simulink model "walkingRobotRL3D"  (R2020b)
settings: Solver=ode23t  StartTime=0.0  StopTime=Tf  RelTol=1e-2  EnableMultiTasking=on
PreLoadFcn:
  | robotParametersRL
undefined symbols (not defined in the file): agent, ankleD_pitch_jointMAX, ankleD_pitch_jointMIN, ankleD_roll_jointMAX, ankleD_roll_jointMIN, ankleI_pitch_jointMAX, ankleI_pitch_jointMIN, ankleI_roll_jointMAX, ankleI_roll_jointMIN, getSampleTime, height_plane, hipD_pitch_jointMAX, hipD_pitch_jointMIN, hipD_roll_jointMAX, hipD_roll_jointMIN, hipI_pitch_jointMAX, hipI_pitch_jointMIN, hipI_roll_jointMAX, hipI_roll_jointMIN, init_angs_L, init_angs_R, init_height, joint_damping, joint_limit_damping, joint_limit_stiffness, joint_stiffness, kneeD_jointMAX, kneeD_jointMIN, kneeI_jointMAX, kneeI_jointMIN, lower_leg_I0, lower_leg_length, lower_leg_mass, lower_leg_x, lower_leg_y, muscle_nominal_length, p10_ankleD_roll, plane_x, plane_y, regulator_type, tau, Tf, torso_height, torso_length, torso_offset_x, torso_offset_z, torso_width, torso_x, torso_y, torso_z, Ts, upper_leg_I0, upper_leg_length, upper_leg_mass, upper_leg_x, upper_leg_y, v10_ankleD_pitch, v10_ankleD_roll, v10_ankleI_pitch, v10_ankleI_roll ... (+41)
libraries: sm_lib x222, simulink x183, nesl_utility x130, walkingRobotUtils x69, rllib x2
(part 1 of 24)
settings Model: Creator=scastro  LastModifiedBy=eri53
settings SolverCC: ZeroCrossAlgorithm=Adaptive
settings DataIOCC: SaveOutput=off  SignalLogging=off  DSMLogging=off  SaveTime=off  ReturnWorkspaceOutputs=off  OutputTimes=0:0.01:10  Refine=2
settings OptimizationCC: LifeSpan=inf
settings DebuggingCC: MaxConsecutiveZCsMsg=warning  IgnoredZcDiagnostic=none  AllowSymbolicDim=off  SFUnexpectedBacktrackingDiag=warning  SFNoUnconditionalDefaultTransitionDiag=warning  SFExecutionAtInitializationDiag=none  UnitsInconsistencyMsg=none  ArithmeticOperatorsInVariantConditions=warning
settings SFSimCC: SimUseLocalCustomCode=off  CustomCodeUndefinedFunction=UseInterfaceOnly
settings RTWCC: RTWUseLocalCustomCode=off
settings CodeAppCC: StateflowObjectComments=on
settings GRTTargetCC: TargetLangStandard=C89/C90 (ANSI)
settings ConfigComp: CovMetricSettings=dw  CovSaveCumulativeToWorkspaceVar=on  CovSaveSingleToWorkspaceVar=on  CovExternalEMLEnable=off  CovSFcnEnable=off
settings SimscapeCC: SimscapeNormalizeSystem=off  SimscapeLogOpenViewer=on  SimscapeLogLimitData=off  SimscapeLogDataHistory=10000
settings ConfigurationSet: Description=SimMechanics 2G
settings DiagnosticsConfigSet: SimMechanicsRigidlyBoundBlock=none
settings ExplorerConfigSet: InternalSimMechanicsExplorerSettings="<ExplorerConfiguration><canonicalview>default</canonicalview><AnimationSetting><BasePlaybackSpeed>1.0</BasePlaybackSpeed><PlaybackSpeedFactor>1.0</PlaybackSpeedFactor></AnimationSetting><TilePanel><TileInfo><Tiles Columns=\"1\" Count=\"1\" Rows=\"1\"><Column Weight=\"1\"/><Row Weight=\"1\"/><Tile Height=\"1\" Width=\"1\" X=\"0\" Y=\"0\"/></Tiles></TileInfo><SceneInfo><SceneViewer><BGColor><R>0.60000002384185791</R><G>0.60000002384185791</G><B>0.60000002384185791</B></BGColor><Camera><DoPerspective>off</DoPerspective><Position><X>8.85055587658612453</X><Y>-7.80751437224638067</Y><Z>7.43266399890212259</Z></Position><Center><X>2.77794058095722196</X><Y>0.225775596241813759</Y><Z>-0.252680675913408259</Z></Center><Up><X>-0.335329266167064488</X><Y>0.506481739462631531</Y><Z>0.79437430147428989</Z></Up><ViewLimDist>1</ViewLimDist><YLim>1.59312668712743077</YLim><XLim>2.57988071665439289</XLim></Camera></SceneViewer></SceneInfo></TilePanel><MechEditorPanel><Cameras/><GfxPanelCameraMap/><VideoCreator><PlaybackSpeedRatio>1.0</PlaybackSpeedRatio><FrameRate>30</FrameRate><VideoFormat>Motion JPEG AVI</VideoFormat><FrameSize>auto</FrameSize></VideoCreator></MechEditorPanel></ExplorerConfiguration>"

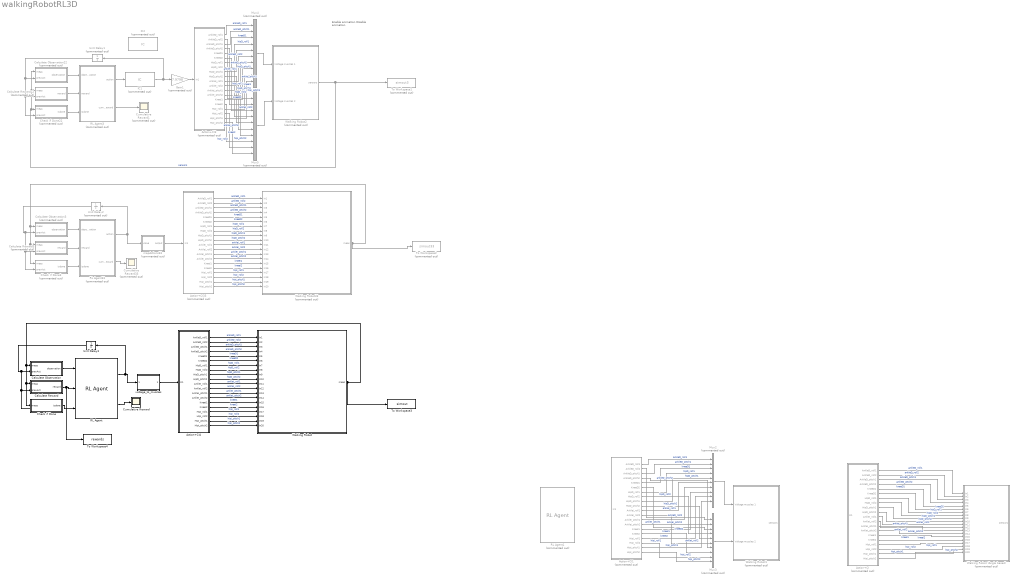
== system walkingRobotRL3D ==
  note: Enable animation
      |
      | Disable animation
  Action+CI : Subsystem  Commented=on
  Action+CI1 : Subsystem  Commented=on
  Action+CI3 : Subsystem  Commented=on
  Action+CI33 : Subsystem  Commented=on
  Action+CI4 : Subsystem
  Calculate Observation : Subsystem
  Calculate Observation22 : Subsystem  Commented=on
  Calculate Observation3 : Subsystem  Commented=on
  Calculate Reward : Subsystem
  Calculate Reward22 : Subsystem  Commented=on
  Calculate Reward3 : Subsystem  Commented=on
  Check if Done : Subsystem
  Check if Done22 : Subsystem  Commented=on
  Check if Done3 : Subsystem  Commented=on
  Cumulative Reward : Scope
  Cumulative Reward1 : Scope  Commented=on
  Cumulative Reward33 : Scope  Commented=on
  Gain1 : Gain  Commented=on  Gain=7.9798
  IC1 : InitialCondition  Commented=on  Value=[v10_ankleD_roll v20_ankleD_roll v10_ankleD_pitch v20_ankleD_pitch v10_kneeD v20_kneeD v10_hipD_roll v20_hipD_roll v10_hipD_pitch v20_hipD_pitch v10_ankleI_roll v20_ankleI_roll v10_ankleI_pitch v20_ankleI_pitch v10_kneeI v20_kneeI v10_hipI_roll v20_hipI_roll v10_hipI_pitch v20_hipI_pitch]'
  IC2 : InitialCondition  Commented=on  Value=(1/7.9798)*[v10_ankleD_roll v20_ankleD_roll v10_ankleD_pitch v20_ankleD_pitch v10_kneeD v20_kneeD v10_hipD_roll v20_hipD_roll v10_hipD_pitch v20_hipD_pitch v10_ankleI_roll v20_ankleI_roll v10_ankleI_pitch v20_ankleI_pitch v10_kneeI v20_kneeI v10_hipI_roll v20_hipI_roll v10_hipI_pitch v20_hipI_pitch]'
  Mux{2..5} (4 alike) : Mux  Commented=on  Inputs=10
  RL Agent : rllib/RL Agent  Agent=agent  ProvideReward=on  ProvideIsDone=on  ProvideCumRwd=on  TreatAsDirectFeedthrough=on  CollectLoggedSignals=on  CollectModelStates=on
  RL Agent1 : rllib/RL Agent  Commented=on  Agent=agent  ProvideReward=on  ProvideIsDone=on  ProvideCumRwd=on  TreatAsDirectFeedthrough=on  CollectLoggedSignals=on  CollectModelStates=on
      settings: SourceProductName=Reinforcement Learning
  RL Agent3 : Subsystem  Commented=on  mask(RL Agent){Agent=agent, ProvideReward=on, ProvideIsDone=on, ProvideCumRwd=on, TreatAsDirectFeedthrough=on, CollectLoggedSignals=on, CollectModelStates=on}
      mask prompts: Agent "rl:block:RLAgentAgentPrompt"; ProvideReward "rl:block:RLAgentProvideRewardPrompt"; ProvideIsDone "rl:block:RLAgentProvideIsDonePrompt"; ProvideCumRwd "rl:block:RLAgentProvideCumRwdPrompt"; TreatAsDirectFeedthrough "rl:block:RLAgentDirectFeedthroughPrompt"; CollectLoggedSignals "rl:block:RLAgentCollectLoggedSignalsPrompt"; CollectModelStates "rl:block:RLAgentCollectModelStatesPrompt"
      mask help: rl:block:RLAgentDescription
      mask init:
      | agentmaskinit(gcb);
      mask Help: eval('rl.util.guihelp(''rlAgentBlock'')')
      mask DialogControl BDCollapsible Prompt: Block Diagram
      mask DialogControl AgentGroup Prompt: rl:block:RLAgentAgentGroupPrompt
      mask DialogControl Agent Prompt: Agent object
      mask DialogControl Agent Tooltip: rl:block:RLAgentAgentTooltip
      mask DialogControl PortGroup Prompt: rl:block:RLAgentPortsGroupPrompt
      mask DialogControl ProvideReward Prompt: Provide reward signal
      mask DialogControl ProvideReward Tooltip: rl:block:RLAgentProvideRewardTooltip
      mask DialogControl ProvideIsDone Prompt: Provide isdone signal
      mask DialogControl ProvideIsDone Tooltip: rl:block:RLAgentProvideIsDoneTooltip
      mask DialogControl ProvideCumRwd Prompt: Output cumulative reward signal
      mask DialogControl ProvideCumRwd Tooltip: rl:block:RLAgentProvideCumRwdTooltip
      mask DialogControl DirectFeedThroughGroup Prompt: rl:block:RLAgentDirectFeedthroughGroupPrompt
      mask DialogControl TreatAsDirectFeedthrough Prompt: Treat inputs as direct feedthrough
      mask DialogControl TreatAsDirectFeedthrough Tooltip: rl:block:RLAgentDirectFeedthroughTooltip
      mask DialogControl DataGroup Prompt: rl:block:RLAgentDataGroupPrompt
      mask DialogControl CollectLoggedSignals Prompt: Provide logged signals to agent
      mask DialogControl CollectLoggedSignals Tooltip: rl:block:RLAgentCollectLoggedSignalsTooltip
      mask DialogControl CollectModelStates Prompt: Provide model states to agent
      mask DialogControl CollectModelStates Tooltip: rl:block:RLAgentCollectModelStatesTooltip
  RL Agent33 : Subsystem  Commented=on  mask(RL Agent){Agent=agent, ProvideReward=on, ProvideIsDone=on, ProvideCumRwd=on, TreatAsDirectFeedthrough=on, CollectLoggedSignals=on, CollectModelStates=on}
      mask prompts: Agent "rl:block:RLAgentAgentPrompt"; ProvideReward "rl:block:RLAgentProvideRewardPrompt"; ProvideIsDone "rl:block:RLAgentProvideIsDonePrompt"; ProvideCumRwd "rl:block:RLAgentProvideCumRwdPrompt"; TreatAsDirectFeedthrough "rl:block:RLAgentDirectFeedthroughPrompt"; CollectLoggedSignals "rl:block:RLAgentCollectLoggedSignalsPrompt"; CollectModelStates "rl:block:RLAgentCollectModelStatesPrompt"
      mask help: rl:block:RLAgentDescription
      mask init:
      | agentmaskinit(gcb);
      mask Help: eval('rl.util.guihelp(''rlAgentBlock'')')
      mask DialogControl BDCollapsible Prompt: Block Diagram
      mask DialogControl AgentGroup Prompt: rl:block:RLAgentAgentGroupPrompt
      mask DialogControl Agent Prompt: Agent object
      mask DialogControl Agent Tooltip: rl:block:RLAgentAgentTooltip
      mask DialogControl PortGroup Prompt: rl:block:RLAgentPortsGroupPrompt
      mask DialogControl ProvideReward Prompt: Provide reward signal
      mask DialogControl ProvideReward Tooltip: rl:block:RLAgentProvideRewardTooltip
      mask DialogControl ProvideIsDone Prompt: Provide isdone signal
      mask DialogControl ProvideIsDone Tooltip: rl:block:RLAgentProvideIsDoneTooltip
      mask DialogControl ProvideCumRwd Prompt: Output cumulative reward signal
      mask DialogControl ProvideCumRwd Tooltip: rl:block:RLAgentProvideCumRwdTooltip
      mask DialogControl DirectFeedThroughGroup Prompt: rl:block:RLAgentDirectFeedthroughGroupPrompt
      mask DialogControl TreatAsDirectFeedthrough Prompt: Treat inputs as direct feedthrough
      mask DialogControl TreatAsDirectFeedthrough Tooltip: rl:block:RLAgentDirectFeedthroughTooltip
      mask DialogControl DataGroup Prompt: rl:block:RLAgentDataGroupPrompt
      mask DialogControl CollectLoggedSignals Prompt: Provide logged signals to agent
      mask DialogControl CollectLoggedSignals Tooltip: rl:block:RLAgentCollectLoggedSignalsTooltip
      mask DialogControl CollectModelStates Prompt: Provide model states to agent
      mask DialogControl CollectModelStates Tooltip: rl:block:RLAgentCollectModelStatesTooltip
  To Workspace1 : ToWorkspace  Commented=on  VariableName=simout3  SaveFormat=Timeseries  SampleTime=-1
  To Workspace2 : ToWorkspace  Commented=on  VariableName=simout33  SaveFormat=Timeseries  SampleTime=-1
  To Workspace3 : ToWorkspace  VariableName=simout  SaveFormat=Timeseries  SampleTime=-1
  To Workspace4 : ToWorkspace  VariableName=rewards  SaveFormat=Timeseries  SampleTime=-1
  Unit Delay1 : UnitDelay  Commented=on  SampleTime=-1  HasFrameUpgradeWarning=on
  Unit Delay2 : UnitDelay  Commented=on  SampleTime=-1  HasFrameUpgradeWarning=on
  Unit Delay3 : UnitDelay  SampleTime=-1  HasFrameUpgradeWarning=on
  Walking Robot : Subsystem
  Walking Robot (Angle based) : Subsystem  Commented=on
      mask Display: image('C:\Users\eri53\Desktop\MASTER\TFM\WALKING ROBOT\OpenLoop(10DoF)\IconosSimulink\lowerLimbRobot.PNG'); % Use "Edit Image" on toolstrip to change.
  Walking Robot1 : Subsystem  Commented=on
      mask Display: image('C:\Users\eri53\Desktop\MASTER\TFM\WALKING ROBOT\OpenLoop(10DoF)\IconosSimulink\lowerLimbRobot.PNG'); % Use "Edit Image" on toolstrip to change.
  Walking Robot2 : Subsystem  Commented=on
  Walking Robot33 : Subsystem  Commented=on
  mapActions33 : MATLAB Function  Commented=on  TreatAsAtomicUnit=on
  voltage_to_muscles : MATLAB Function  TreatAsAtomicUnit=on
  wires:
  Action+CI1/4(AnkleD_pitch2) -> Mux3/2  "ankleD_pitch2"
  Action+CI1/15(KneeI1) -> Mux2/8  "kneeI1"
  Action+CI1/18(HipI_roll2) -> Mux3/9  "hipI_roll2"
  Action+CI1/3(AnkleD_pitch1) -> Mux2/2  "ankleD_pitch1"
  Action+CI1/20(HipI_pitch2) -> Mux3/10  "hipI_pitch2"
  Action+CI1/16(KneeI2) -> Mux3/8  "kneeI2"
  Action+CI1/9(HipD_pitch1) -> Mux2/5  "hipD_pitch1"
  Action+CI1/14(AnkleI_pitch2) -> Mux3/7  "ankleI_pitch2"
  Action+CI1/11(AnkleI_roll1) -> Mux2/6  "ankleI_roll1"
  Action+CI1/2(AnkleD_roll2) -> Mux3/1  "ankleD_roll2"
  Action+CI1/1(AnkleD_roll1) -> Mux2/1  "ankleD_roll1"
  Action+CI1/7(HipD_roll1) -> Mux2/4  "hipD_roll1"
  Action+CI1/10(HipD_pitch2) -> Mux3/5  "hipD_pitch2"
  Action+CI1/19(HipI_pitch1) -> Mux2/10  "hipI_pitch1"
  Action+CI1/8(HipD_roll2) -> Mux3/4  "hipD_roll2"
  Action+CI1/17(HipI_roll1) -> Mux2/9  "hipI_roll1"
  Action+CI1/6(KneeD2) -> Mux3/3  "kneeD2"
  Action+CI1/12(AnkleI_roll2) -> Mux3/6  "ankleI_roll2"
  Action+CI1/13(AnkleI_pitch1) -> Mux2/7  "ankleI_pitch1"
  Action+CI1/5(KneeD1) -> Mux2/3  "kneeD1"
  Mux3/1 -> Walking Robot1/2(Voltage muscles 2)
  Mux2/1 -> Walking Robot1/1(Voltage muscles 1)
  Action+CI/1(AnkleD_roll1) -> Walking Robot (Angle based)/1(In1)  "ankleD_roll1"
  Action+CI/2(AnkleD_roll2) -> Walking Robot (Angle based)/2(In2)  "ankleD_roll2"
  Action+CI/3(AnkleD_pitch1) -> Walking Robot (Angle based)/3(In3)  "ankleD_pitch1"
  Action+CI/4(AnkleD_pitch2) -> Walking Robot (Angle based)/4(In4)  "ankleD_pitch2"
  Action+CI/5(KneeD1) -> Walking Robot (Angle based)/5(In5)  "kneeD1"
  Action+CI/6(KneeD2) -> Walking Robot (Angle based)/6(In6)  "kneeD2"
  Action+CI/7(HipD_roll1) -> Walking Robot (Angle based)/7(In7)  "hipD_roll1"
  Action+CI/8(HipD_roll2) -> Walking Robot (Angle based)/8(In8)  "hipD_roll2"
  Action+CI/9(HipD_pitch1) -> Walking Robot (Angle based)/9(In9)  "hipD_pitch1"
  Action+CI/10(HipD_pitch2) -> Walking Robot (Angle based)/10(In10)  "hipD_pitch2"
  Action+CI/11(AnkleI_roll1) -> Walking Robot (Angle based)/11(In11)  "ankleI_roll1"
  Action+CI/12(AnkleI_roll2) -> Walking Robot (Angle based)/12(In12)  "ankleI_roll2"
  Action+CI/13(AnkleI_pitch1) -> Walking Robot (Angle based)/13(In13)  "ankleI_pitch1"
  Action+CI/14(AnkleI_pitch2) -> Walking Robot (Angle based)/14(In14)  "ankleI_pitch2"
  Action+CI/15(KneeI1) -> Walking Robot (Angle based)/15(In15)  "kneeI1"
  Action+CI/16(KneeI2) -> Walking Robot (Angle based)/16(In16)  "kneeI2"
  Action+CI/17(HipI_roll1) -> Walking Robot (Angle based)/17(In17)  "hipI_roll1"
  Action+CI/18(HipI_roll2) -> Walking Robot (Angle based)/18(In18)  "hipI_roll2"
  Action+CI/19(HipI_pitch1) -> Walking Robot (Angle based)/19(In19)  "hipI_pitch1"
  Action+CI/20(HipI_pitch2) -> Walking Robot (Angle based)/20(In20)  "hipI_pitch2"
  Action+CI3/12(AnkleI_roll2) -> Mux5/6  "ankleI_roll2"
  Unit Delay1/1 -> Check if Done22/2(prevAct), Calculate Reward22/2(prevAct), Calculate Observation22/2(prevAct)
  Action+CI3/9(HipD_pitch1) -> Mux4/5  "hipD_pitch1"
  Action+CI3/8(HipD_roll2) -> Mux5/4  "hipD_roll2"
  Gain1/1 -> Action+CI3/1(In1)
  IC1/1 -> Unit Delay1/1, Gain1/1
  Action+CI3/3(AnkleD_pitch1) -> Mux4/2  "ankleD_pitch1"
  Action+CI3/7(HipD_roll1) -> Mux4/4  "hipD_roll1"
  Action+CI3/17(HipI_roll1) -> Mux4/9  "hipI_roll1"
  Action+CI3/20(HipI_pitch2) -> Mux5/10  "hipI_pitch2"
  Action+CI3/16(KneeI2) -> Mux5/8  "kneeI2"
  RL Agent3/2(cumulative_reward) -> Cumulative Reward1/1
  Action+CI3/14(AnkleI_pitch2) -> Mux5/7  "ankleI_pitch2"
  Action+CI3/11(AnkleI_roll1) -> Mux4/6  "ankleI_roll1"
  Mux5/1 -> Walking Robot2/2(Voltage muscles 2)
  Action+CI3/10(HipD_pitch2) -> Mux5/5  "hipD_pitch2"
  Action+CI3/18(HipI_roll2) -> Mux5/9  "hipI_roll2"
  Action+CI3/2(AnkleD_roll2) -> Mux5/1  "ankleD_roll2"
  Mux4/1 -> Walking Robot2/1(Voltage muscles 1)
  Calculate Observation22/1(observation) -> RL Agent3/1(observation)
  Action+CI3/13(AnkleI_pitch1) -> Mux4/7  "ankleI_pitch1"
  Walking Robot2/1(sensors) -> Calculate Observation22/1(meas), Calculate Reward22/1(meas), Check if Done22/1(meas), To Workspace1/1  "sensors"
  Action+CI3/6(KneeD2) -> Mux5/3  "kneeD2"
  Action+CI3/5(KneeD1) -> Mux4/3  "kneeD1"
  Check if Done22/1(isdone) -> RL Agent3/3(isdone)
  Action+CI3/19(HipI_pitch1) -> Mux4/10  "hipI_pitch1"
  Calculate Reward22/1(reward) -> RL Agent3/2(reward)
  RL Agent3/1(action) -> IC1/1
  Action+CI3/4(AnkleD_pitch2) -> Mux5/2  "ankleD_pitch2"
  Action+CI3/15(KneeI1) -> Mux4/8  "kneeI1"
  Action+CI3/1(AnkleD_roll1) -> Mux4/1  "ankleD_roll1"
  Action+CI33/1(AnkleD_roll1) -> Walking Robot33/1(In1)  "ankleD_roll1"
  Action+CI33/2(AnkleD_roll2) -> Walking Robot33/2(In2)  "ankleD_roll2"
  Action+CI33/3(AnkleD_pitch1) -> Walking Robot33/3(In3)  "ankleD_pitch1"
  Action+CI33/4(AnkleD_pitch2) -> Walking Robot33/4(In4)  "ankleD_pitch2"
  Action+CI33/5(KneeD1) -> Walking Robot33/5(In5)  "kneeD1"
  Action+CI33/6(KneeD2) -> Walking Robot33/6(In6)  "kneeD2"
  Action+CI33/7(HipD_roll1) -> Walking Robot33/7(In7)  "hipD_roll1"
  Action+CI33/8(HipD_roll2) -> Walking Robot33/8(In8)  "hipD_roll2"
  Action+CI33/9(HipD_pitch1) -> Walking Robot33/9(In9)  "hipD_pitch1"
  Action+CI33/10(HipD_pitch2) -> Walking Robot33/10(In10)  "hipD_pitch2"
  Action+CI33/11(AnkleI_roll1) -> Walking Robot33/11(In11)  "ankleI_roll1"
  Action+CI33/12(AnkleI_roll2) -> Walking Robot33/12(In12)  "ankleI_roll2"
  Action+CI33/13(AnkleI_pitch1) -> Walking Robot33/13(In13)  "ankleI_pitch1"
  Action+CI33/14(AnkleI_pitch2) -> Walking Robot33/14(In14)  "ankleI_pitch2"
  Action+CI33/15(KneeI1) -> Walking Robot33/15(In15)  "kneeI1"
  Action+CI33/16(KneeI2) -> Walking Robot33/16(In16)  "kneeI2"
  Action+CI33/17(HipI_roll1) -> Walking Robot33/17(In17)  "hipI_roll1"
  Action+CI33/18(HipI_roll2) -> Walking Robot33/18(In18)  "hipI_roll2"
  Action+CI33/19(HipI_pitch1) -> Walking Robot33/19(In19)  "hipI_pitch1"
  Action+CI33/20(HipI_pitch2) -> Walking Robot33/20(In20)  "hipI_pitch2"
  RL Agent33/2(cumulative_reward) -> Cumulative Reward33/1
  Calculate Observation3/1(observation) -> RL Agent33/1(observation)
  Calculate Reward3/1(reward) -> RL Agent33/2(reward)
  Check if Done3/1(isdone) -> RL Agent33/3(isdone)
  RL Agent33/1(action) -> Unit Delay2/1, mapActions33/1(value)
  Walking Robot33/1(meas) -> Check if Done3/1(meas), Calculate Reward3/1(meas), Calculate Observation3/1(meas), To Workspace2/1
  Unit Delay2/1 -> Check if Done3/2(prevAct), Calculate Reward3/2(prevAct), Calculate Observation3/2(prevAct)
  mapActions33/1(output) -> Action+CI33/1(In1)
  voltage_to_muscles/1(mapped_actions) -> Action+CI4/1(In1)
  Unit Delay3/1 -> Calculate Reward/2(prevAct), Calculate Observation/2(prevAct)
  Action+CI4/10(HipD_pitch2) -> Walking Robot/10(In10)  "hipD_pitch2"
  Action+CI4/9(HipD_pitch1) -> Walking Robot/9(In9)  "hipD_pitch1"
  Walking Robot/1(meas) -> Check if Done/1(meas), Calculate Reward/1(meas), Calculate Observation/1(meas), To Workspace3/1
  Action+CI4/14(AnkleI_pitch2) -> Walking Robot/14(In14)  "ankleI_pitch2"
  Action+CI4/7(HipD_roll1) -> Walking Robot/7(In7)  "hipD_roll1"
  Action+CI4/20(HipI_pitch2) -> Walking Robot/20(In20)  "hipI_pitch2"
  Action+CI4/19(HipI_pitch1) -> Walking Robot/19(In19)  "hipI_pitch1"
  Action+CI4/11(AnkleI_roll1) -> Walking Robot/11(In11)  "ankleI_roll1"
  Action+CI4/13(AnkleI_pitch1) -> Walking Robot/13(In13)  "ankleI_pitch1"
  Action+CI4/16(KneeI2) -> Walking Robot/16(In16)  "kneeI2"
  Action+CI4/17(HipI_roll1) -> Walking Robot/17(In17)  "hipI_roll1"
  Action+CI4/15(KneeI1) -> Walking Robot/15(In15)  "kneeI1"
  Action+CI4/6(KneeD2) -> Walking Robot/6(In6)  "kneeD2"
  Action+CI4/8(HipD_roll2) -> Walking Robot/8(In8)  "hipD_roll2"
  Action+CI4/18(HipI_roll2) -> Walking Robot/18(In18)  "hipI_roll2"
  Action+CI4/2(AnkleD_roll2) -> Walking Robot/2(In2)  "ankleD_roll2"
  Action+CI4/5(KneeD1) -> Walking Robot/5(In5)  "kneeD1"
  Action+CI4/1(AnkleD_roll1) -> Walking Robot/1(In1)  "ankleD_roll1"
  Action+CI4/12(AnkleI_roll2) -> Walking Robot/12(In12)  "ankleI_roll2"
  Action+CI4/3(AnkleD_pitch1) -> Walking Robot/3(In3)  "ankleD_pitch1"
  Action+CI4/4(AnkleD_pitch2) -> Walking Robot/4(In4)  "ankleD_pitch2"
  Calculate Observation/1(observation) -> RL Agent/1
  Calculate Reward/1(reward) -> To Workspace4/1, RL Agent/2
  Check if Done/1(isdone) -> RL Agent/3
  RL Agent/1 -> Unit Delay3/1, voltage_to_muscles/1(actions)
  RL Agent/2 -> Cumulative Reward/1

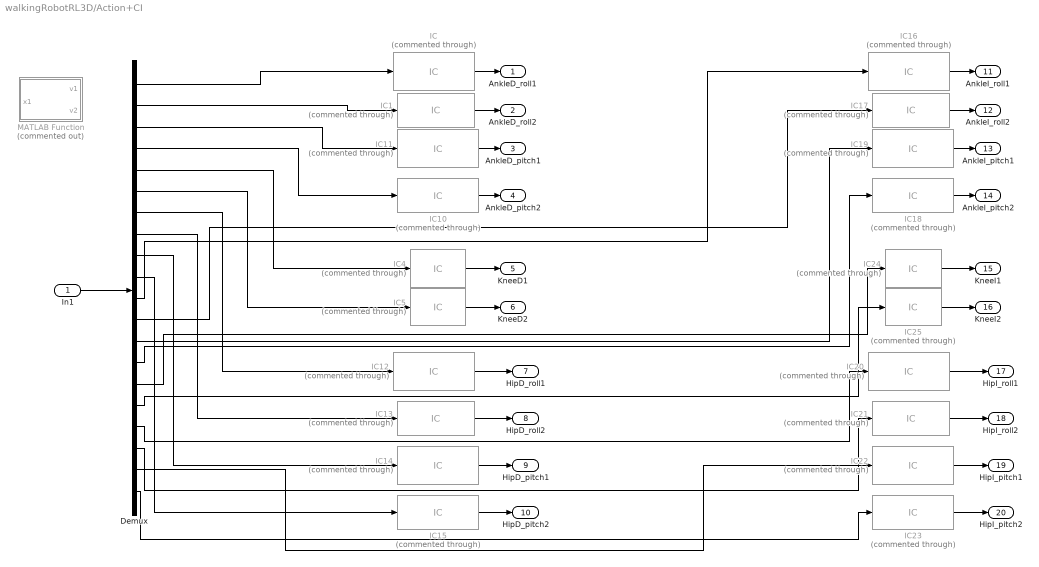
== system walkingRobotRL3D/Action+CI ==
  In1 : Inport
  Demux : Demux  Outputs=20
  IC : InitialCondition  Commented=through  Value=v10_ankleD_roll
  IC1 : InitialCondition  Commented=through  Value=v20_ankleD_roll
  IC10 : InitialCondition  Commented=through  Value=v20_ankleD_pitch
  IC11 : InitialCondition  Commented=through  Value=v10_ankleD_pitch
  IC12 : InitialCondition  Commented=through  Value=v10_hipD_roll
  IC13 : InitialCondition  Commented=through  Value=v20_hipD_roll
  IC14 : InitialCondition  Commented=through  Value=v10_hipD_pitch
  IC15 : InitialCondition  Commented=through  Value=v20_hipD_pitch
  IC16 : InitialCondition  Commented=through  Value=v10_ankleI_roll
  IC17 : InitialCondition  Commented=through  Value=v20_ankleI_roll
  IC18 : InitialCondition  Commented=through  Value=v20_ankleI_pitch
  IC19 : InitialCondition  Commented=through  Value=v10_ankleI_pitch
  IC20 : InitialCondition  Commented=through  Value=v10_hipI_roll
  IC21 : InitialCondition  Commented=through  Value=v20_hipI_roll
  IC22 : InitialCondition  Commented=through  Value=v10_hipI_pitch
  IC23 : InitialCondition  Commented=through  Value=v20_hipI_pitch
  IC24 : InitialCondition  Commented=through  Value=v10_kneeI
  IC25 : InitialCondition  Commented=through  Value=v20_kneeI
  IC4 : InitialCondition  Commented=through  Value=v10_kneeD
  IC5 : InitialCondition  Commented=through  Value=v20_kneeD
  MATLAB Function : MATLAB Function  Commented=on  TreatAsAtomicUnit=on
  AnkleD_roll1 : Outport
  AnkleD_roll2 : Outport  Port=2
  AnkleD_pitch1 : Outport  Port=3
  AnkleD_pitch2 : Outport  Port=4
  KneeD1 : Outport  Port=5
  KneeD2 : Outport  Port=6
  HipD_roll1 : Outport  Port=7
  HipD_roll2 : Outport  Port=8
  HipD_pitch1 : Outport  Port=9
  HipD_pitch2 : Outport  Port=10
  AnkleI_roll1 : Outport  Port=11
  AnkleI_roll2 : Outport  Port=12
  AnkleI_pitch1 : Outport  Port=13
  AnkleI_pitch2 : Outport  Port=14
  KneeI1 : Outport  Port=15
  KneeI2 : Outport  Port=16
  HipI_roll1 : Outport  Port=17
  HipI_roll2 : Outport  Port=18
  HipI_pitch1 : Outport  Port=19
  HipI_pitch2 : Outport  Port=20
  wires:
  IC/1 -> AnkleD_roll1/1
  IC1/1 -> AnkleD_roll2/1
  IC4/1 -> KneeD1/1
  IC5/1 -> KneeD2/1
  IC11/1 -> AnkleD_pitch1/1
  IC10/1 -> AnkleD_pitch2/1
  IC12/1 -> HipD_roll1/1
  IC13/1 -> HipD_roll2/1
  IC14/1 -> HipD_pitch1/1
  IC15/1 -> HipD_pitch2/1
  IC22/1 -> HipI_pitch1/1
  IC24/1 -> KneeI1/1
  IC23/1 -> HipI_pitch2/1
  IC20/1 -> HipI_roll1/1
  IC21/1 -> HipI_roll2/1
  IC18/1 -> AnkleI_pitch2/1
  IC25/1 -> KneeI2/1
  IC16/1 -> AnkleI_roll1/1
  IC19/1 -> AnkleI_pitch1/1
  IC17/1 -> AnkleI_roll2/1
  In1/1 -> Demux/1
  Demux/1 -> IC/1
  Demux/2 -> IC1/1
  Demux/3 -> IC11/1
  Demux/4 -> IC10/1
  Demux/5 -> IC4/1
  Demux/6 -> IC5/1
  Demux/7 -> IC12/1
  Demux/8 -> IC13/1
  Demux/9 -> IC14/1
  Demux/10 -> IC15/1
  Demux/11 -> IC16/1
  Demux/12 -> IC17/1
  Demux/13 -> IC19/1
  Demux/14 -> IC18/1
  Demux/15 -> IC24/1
  Demux/16 -> IC25/1
  Demux/17 -> IC20/1
  Demux/18 -> IC21/1
  Demux/19 -> IC22/1
  Demux/20 -> IC23/1

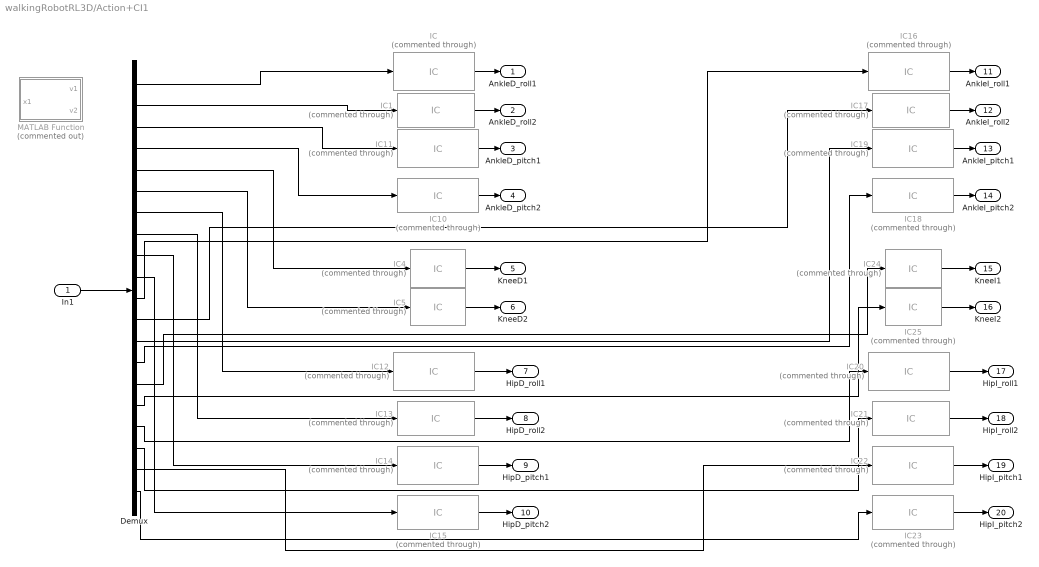
== system walkingRobotRL3D/Action+CI1 ==
  In1 : Inport
  Demux : Demux  Outputs=20
  IC : InitialCondition  Commented=through  Value=v10_ankleD_roll
  IC1 : InitialCondition  Commented=through  Value=v20_ankleD_roll
  IC10 : InitialCondition  Commented=through  Value=v20_ankleD_pitch
  IC11 : InitialCondition  Commented=through  Value=v10_ankleD_pitch
  IC12 : InitialCondition  Commented=through  Value=v10_hipD_roll
  IC13 : InitialCondition  Commented=through  Value=v20_hipD_roll
  IC14 : InitialCondition  Commented=through  Value=v10_hipD_pitch
  IC15 : InitialCondition  Commented=through  Value=v20_hipD_pitch
  IC16 : InitialCondition  Commented=through  Value=v10_ankleI_roll
  IC17 : InitialCondition  Commented=through  Value=v20_ankleI_roll
  IC18 : InitialCondition  Commented=through  Value=v20_ankleI_pitch
  IC19 : InitialCondition  Commented=through  Value=v10_ankleI_pitch
  IC20 : InitialCondition  Commented=through  Value=v10_hipI_roll
  IC21 : InitialCondition  Commented=through  Value=v20_hipI_roll
  IC22 : InitialCondition  Commented=through  Value=v10_hipI_pitch
  IC23 : InitialCondition  Commented=through  Value=v20_hipI_pitch
  IC24 : InitialCondition  Commented=through  Value=v10_kneeI
  IC25 : InitialCondition  Commented=through  Value=v20_kneeI
  IC4 : InitialCondition  Commented=through  Value=v10_kneeD
  IC5 : InitialCondition  Commented=through  Value=v20_kneeD
  MATLAB Function : MATLAB Function  Commented=on  TreatAsAtomicUnit=on
  AnkleD_roll1 : Outport
  AnkleD_roll2 : Outport  Port=2
  AnkleD_pitch1 : Outport  Port=3
  AnkleD_pitch2 : Outport  Port=4
  KneeD1 : Outport  Port=5
  KneeD2 : Outport  Port=6
  HipD_roll1 : Outport  Port=7
  HipD_roll2 : Outport  Port=8
  HipD_pitch1 : Outport  Port=9
  HipD_pitch2 : Outport  Port=10
  AnkleI_roll1 : Outport  Port=11
  AnkleI_roll2 : Outport  Port=12
  AnkleI_pitch1 : Outport  Port=13
  AnkleI_pitch2 : Outport  Port=14
  KneeI1 : Outport  Port=15
  KneeI2 : Outport  Port=16
  HipI_roll1 : Outport  Port=17
  HipI_roll2 : Outport  Port=18
  HipI_pitch1 : Outport  Port=19
  HipI_pitch2 : Outport  Port=20
  wires:
  IC/1 -> AnkleD_roll1/1
  IC1/1 -> AnkleD_roll2/1
  IC4/1 -> KneeD1/1
  IC5/1 -> KneeD2/1
  IC11/1 -> AnkleD_pitch1/1
  IC10/1 -> AnkleD_pitch2/1
  IC12/1 -> HipD_roll1/1
  IC13/1 -> HipD_roll2/1
  IC14/1 -> HipD_pitch1/1
  IC15/1 -> HipD_pitch2/1
  IC22/1 -> HipI_pitch1/1
  IC24/1 -> KneeI1/1
  IC23/1 -> HipI_pitch2/1
  IC20/1 -> HipI_roll1/1
  IC21/1 -> HipI_roll2/1
  IC18/1 -> AnkleI_pitch2/1
  IC25/1 -> KneeI2/1
  IC16/1 -> AnkleI_roll1/1
  IC19/1 -> AnkleI_pitch1/1
  IC17/1 -> AnkleI_roll2/1
  In1/1 -> Demux/1
  Demux/1 -> IC/1
  Demux/2 -> IC1/1
  Demux/3 -> IC11/1
  Demux/4 -> IC10/1
  Demux/5 -> IC4/1
  Demux/6 -> IC5/1
  Demux/7 -> IC12/1
  Demux/8 -> IC13/1
  Demux/9 -> IC14/1
  Demux/10 -> IC15/1
  Demux/11 -> IC16/1
  Demux/12 -> IC17/1
  Demux/13 -> IC19/1
  Demux/14 -> IC18/1
  Demux/15 -> IC24/1
  Demux/16 -> IC25/1
  Demux/17 -> IC20/1
  Demux/18 -> IC21/1
  Demux/19 -> IC22/1
  Demux/20 -> IC23/1

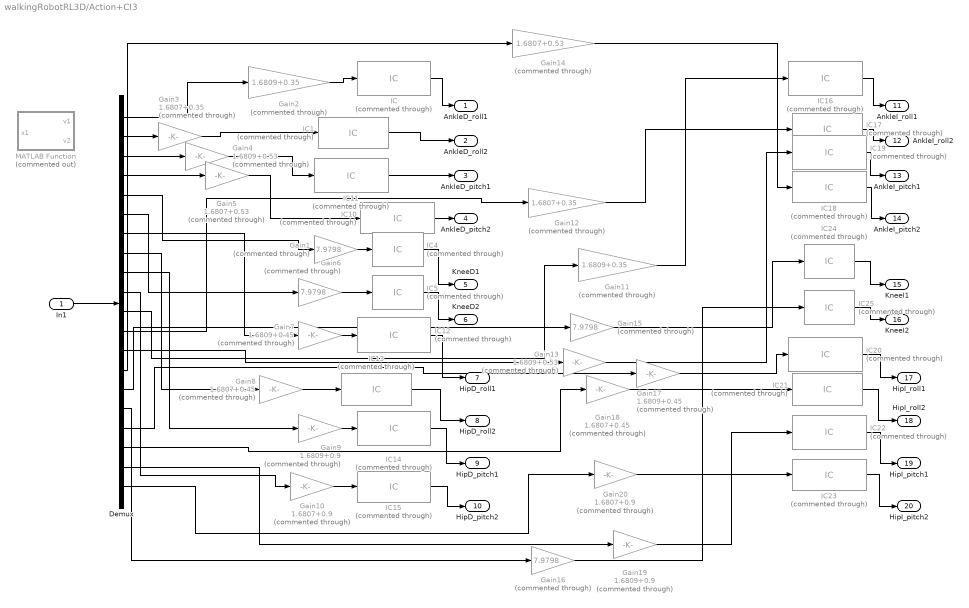
== system walkingRobotRL3D/Action+CI3 ==
  In1 : Inport
  Demux : Demux  Outputs=20
  Gain{1,6,15..16} (4 alike) : Gain  Commented=through  Gain=7.9798
  Gain10 : Gain  Commented=through  Gain=1.6807+0.9
  Gain11 : Gain  Commented=through  Gain=1.6809+0.35
  Gain12 : Gain  Commented=through  Gain=1.6807+0.35
  Gain13 : Gain  Commented=through  Gain=1.6809+0.53
  Gain14 : Gain  Commented=through  Gain=1.6807+0.53
  Gain17 : Gain  Commented=through  Gain=1.6809+0.45
  Gain18 : Gain  Commented=through  Gain=1.6807+0.45
  Gain19 : Gain  Commented=through  Gain=1.6809+0.9
  Gain2 : Gain  Commented=through  Gain=1.6809+0.35
  Gain20 : Gain  Commented=through  Gain=1.6807+0.9
  Gain3 : Gain  Commented=through  Gain=1.6807+0.35
  Gain4 : Gain  Commented=through  Gain=1.6809+0.53
  Gain5 : Gain  Commented=through  Gain=1.6807+0.53
  Gain7 : Gain  Commented=through  Gain=1.6809+0.45
  Gain8 : Gain  Commented=through  Gain=1.6807+0.45
  Gain9 : Gain  Commented=through  Gain=1.6809+0.9
  IC : InitialCondition  Commented=through  Value=v10_ankleD_roll
  IC1 : InitialCondition  Commented=through  Value=v20_ankleD_roll
  IC10 : InitialCondition  Commented=through  Value=v20_ankleD_pitch
  IC11 : InitialCondition  Commented=through  Value=v10_ankleD_pitch
  IC12 : InitialCondition  Commented=through  Value=v10_hipD_roll
  IC13 : InitialCondition  Commented=through  Value=v20_hipD_roll
  IC14 : InitialCondition  Commented=through  Value=v10_hipD_pitch
  IC15 : InitialCondition  Commented=through  Value=v20_hipD_pitch
  IC16 : InitialCondition  Commented=through  Value=v10_ankleI_roll
  IC17 : InitialCondition  Commented=through  Value=v20_ankleI_roll
  IC18 : InitialCondition  Commented=through  Value=v20_ankleI_pitch
  IC19 : InitialCondition  Commented=through  Value=v10_ankleI_pitch
  IC20 : InitialCondition  Commented=through  Value=v10_hipI_roll
  IC21 : InitialCondition  Commented=through  Value=v20_hipI_roll
  IC22 : InitialCondition  Commented=through  Value=v10_hipI_pitch
  IC23 : InitialCondition  Commented=through  Value=v20_hipI_pitch
  IC24 : InitialCondition  Commented=through  Value=v10_kneeI
  IC25 : InitialCondition  Commented=through  Value=v20_kneeI
  IC4 : InitialCondition  Commented=through  Value=v10_kneeD
  IC5 : InitialCondition  Commented=through  Value=v20_kneeD
  MATLAB Function : MATLAB Function  Commented=on  TreatAsAtomicUnit=on
  AnkleD_roll1 : Outport
  AnkleD_roll2 : Outport  Port=2
  AnkleD_pitch1 : Outport  Port=3
  AnkleD_pitch2 : Outport  Port=4
  KneeD1 : Outport  Port=5
  KneeD2 : Outport  Port=6
  HipD_roll1 : Outport  Port=7
  HipD_roll2 : Outport  Port=8
  HipD_pitch1 : Outport  Port=9
  HipD_pitch2 : Outport  Port=10
  AnkleI_roll1 : Outport  Port=11
  AnkleI_roll2 : Outport  Port=12
  AnkleI_pitch1 : Outport  Port=13
  AnkleI_pitch2 : Outport  Port=14
  KneeI1 : Outport  Port=15
  KneeI2 : Outport  Port=16
  HipI_roll1 : Outport  Port=17
  HipI_roll2 : Outport  Port=18
  HipI_pitch1 : Outport  Port=19
  HipI_pitch2 : Outport  Port=20
  wires:
  IC/1 -> AnkleD_roll1/1
  IC1/1 -> AnkleD_roll2/1
  IC4/1 -> KneeD1/1
  IC5/1 -> KneeD2/1
  IC11/1 -> AnkleD_pitch1/1
  IC10/1 -> AnkleD_pitch2/1
  IC12/1 -> HipD_roll1/1
  IC13/1 -> HipD_roll2/1
  IC14/1 -> HipD_pitch1/1
  IC15/1 -> HipD_pitch2/1
  IC22/1 -> HipI_pitch1/1
  IC24/1 -> KneeI1/1
  IC23/1 -> HipI_pitch2/1
  IC20/1 -> HipI_roll1/1
  IC21/1 -> HipI_roll2/1
  IC18/1 -> AnkleI_pitch2/1
  IC25/1 -> KneeI2/1
  IC16/1 -> AnkleI_roll1/1
  IC19/1 -> AnkleI_pitch1/1
  IC17/1 -> AnkleI_roll2/1
  In1/1 -> Demux/1
  Demux/1 -> Gain2/1
  Demux/2 -> Gain3/1
  Demux/3 -> Gain4/1
  Demux/4 -> Gain5/1
  Demux/5 -> Gain1/1
  Demux/6 -> Gain6/1
  Demux/7 -> Gain7/1
  Demux/8 -> Gain8/1
  Demux/9 -> Gain9/1
  Demux/10 -> Gain10/1
  Demux/11 -> Gain11/1
  Demux/12 -> Gain12/1
  Demux/13 -> Gain13/1
  Demux/14 -> Gain14/1
  Demux/15 -> Gain15/1
  Demux/16 -> Gain16/1
  Demux/17 -> Gain17/1
  Demux/18 -> Gain18/1
  Demux/19 -> Gain19/1
  Demux/20 -> Gain20/1
  Gain2/1 -> IC/1
  Gain3/1 -> IC1/1
  Gain4/1 -> IC11/1
  Gain5/1 -> IC10/1
  Gain1/1 -> IC4/1
  Gain6/1 -> IC5/1
  Gain7/1 -> IC12/1
  Gain8/1 -> IC13/1
  Gain9/1 -> IC14/1
  Gain10/1 -> IC15/1
  Gain11/1 -> IC16/1
  Gain12/1 -> IC17/1
  Gain13/1 -> IC19/1
  Gain14/1 -> IC18/1
  Gain15/1 -> IC24/1
  Gain16/1 -> IC25/1
  Gain17/1 -> IC20/1
  Gain18/1 -> IC21/1
  Gain19/1 -> IC22/1
  Gain20/1 -> IC23/1

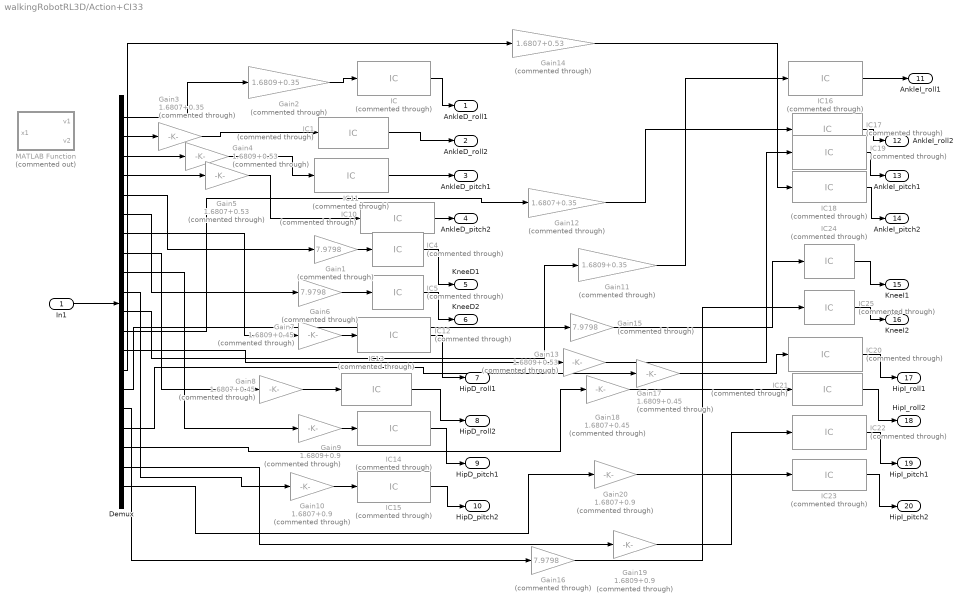
== system walkingRobotRL3D/Action+CI33 ==
  In1 : Inport
  Demux : Demux  Outputs=20
  Gain{1,6,15..16} (4 alike) : Gain  Commented=through  Gain=7.9798
  Gain10 : Gain  Commented=through  Gain=1.6807+0.9
  Gain11 : Gain  Commented=through  Gain=1.6809+0.35
  Gain12 : Gain  Commented=through  Gain=1.6807+0.35
  Gain13 : Gain  Commented=through  Gain=1.6809+0.53
  Gain14 : Gain  Commented=through  Gain=1.6807+0.53
  Gain17 : Gain  Commented=through  Gain=1.6809+0.45
  Gain18 : Gain  Commented=through  Gain=1.6807+0.45
  Gain19 : Gain  Commented=through  Gain=1.6809+0.9
  Gain2 : Gain  Commented=through  Gain=1.6809+0.35
  Gain20 : Gain  Commented=through  Gain=1.6807+0.9
  Gain3 : Gain  Commented=through  Gain=1.6807+0.35
  Gain4 : Gain  Commented=through  Gain=1.6809+0.53
  Gain5 : Gain  Commented=through  Gain=1.6807+0.53
  Gain7 : Gain  Commented=through  Gain=1.6809+0.45
  Gain8 : Gain  Commented=through  Gain=1.6807+0.45
  Gain9 : Gain  Commented=through  Gain=1.6809+0.9
  IC : InitialCondition  Commented=through  Value=v10_ankleD_roll
  IC1 : InitialCondition  Commented=through  Value=v20_ankleD_roll
  IC10 : InitialCondition  Commented=through  Value=v20_ankleD_pitch
  IC11 : InitialCondition  Commented=through  Value=v10_ankleD_pitch
  IC12 : InitialCondition  Commented=through  Value=v10_hipD_roll
  IC13 : InitialCondition  Commented=through  Value=v20_hipD_roll
  IC14 : InitialCondition  Commented=through  Value=v10_hipD_pitch
  IC15 : InitialCondition  Commented=through  Value=v20_hipD_pitch
  IC16 : InitialCondition  Commented=through  Value=v10_ankleI_roll
  IC17 : InitialCondition  Commented=through  Value=v20_ankleI_roll
  IC18 : InitialCondition  Commented=through  Value=v20_ankleI_pitch
  IC19 : InitialCondition  Commented=through  Value=v10_ankleI_pitch
  IC20 : InitialCondition  Commented=through  Value=v10_hipI_roll
  IC21 : InitialCondition  Commented=through  Value=v20_hipI_roll
  IC22 : InitialCondition  Commented=through  Value=v10_hipI_pitch
  IC23 : InitialCondition  Commented=through  Value=v20_hipI_pitch
  IC24 : InitialCondition  Commented=through  Value=v10_kneeI
  IC25 : InitialCondition  Commented=through  Value=v20_kneeI
  IC4 : InitialCondition  Commented=through  Value=v10_kneeD
  IC5 : InitialCondition  Commented=through  Value=v20_kneeD
  MATLAB Function : MATLAB Function  Commented=on  TreatAsAtomicUnit=on
  AnkleD_roll1 : Outport
  AnkleD_roll2 : Outport  Port=2
  AnkleD_pitch1 : Outport  Port=3
  AnkleD_pitch2 : Outport  Port=4
  KneeD1 : Outport  Port=5
  KneeD2 : Outport  Port=6
  HipD_roll1 : Outport  Port=7
  HipD_roll2 : Outport  Port=8
  HipD_pitch1 : Outport  Port=9
  HipD_pitch2 : Outport  Port=10
  AnkleI_roll1 : Outport  Port=11
  AnkleI_roll2 : Outport  Port=12
  AnkleI_pitch1 : Outport  Port=13
  AnkleI_pitch2 : Outport  Port=14
  KneeI1 : Outport  Port=15
  KneeI2 : Outport  Port=16
  HipI_roll1 : Outport  Port=17
  HipI_roll2 : Outport  Port=18
  HipI_pitch1 : Outport  Port=19
  HipI_pitch2 : Outport  Port=20
  wires:
  IC/1 -> AnkleD_roll1/1
  IC1/1 -> AnkleD_roll2/1
  IC4/1 -> KneeD1/1
  IC5/1 -> KneeD2/1
  IC11/1 -> AnkleD_pitch1/1
  IC10/1 -> AnkleD_pitch2/1
  IC12/1 -> HipD_roll1/1
  IC13/1 -> HipD_roll2/1
  IC14/1 -> HipD_pitch1/1
  IC15/1 -> HipD_pitch2/1
  IC22/1 -> HipI_pitch1/1
  IC24/1 -> KneeI1/1
  IC23/1 -> HipI_pitch2/1
  IC20/1 -> HipI_roll1/1
  IC21/1 -> HipI_roll2/1
  IC18/1 -> AnkleI_pitch2/1
  IC25/1 -> KneeI2/1
  IC16/1 -> AnkleI_roll1/1
  IC19/1 -> AnkleI_pitch1/1
  IC17/1 -> AnkleI_roll2/1
  In1/1 -> Demux/1
  Demux/1 -> Gain2/1
  Demux/2 -> Gain3/1
  Demux/3 -> Gain4/1
  Demux/4 -> Gain5/1
  Demux/7 -> Gain7/1
  Demux/8 -> Gain8/1
  Demux/11 -> Gain11/1
  Demux/12 -> Gain12/1
  Demux/13 -> Gain13/1
  Demux/14 -> Gain14/1
  Demux/15 -> Gain15/1
  Demux/16 -> Gain16/1
  Demux/17 -> Gain17/1
  Demux/18 -> Gain18/1
  Demux/19 -> Gain19/1
  Demux/20 -> Gain20/1
  Gain2/1 -> IC/1
  Gain3/1 -> IC1/1
  Gain4/1 -> IC11/1
  Gain5/1 -> IC10/1
  Gain1/1 -> IC4/1
  Gain6/1 -> IC5/1
  Gain7/1 -> IC12/1
  Gain8/1 -> IC13/1
  Gain9/1 -> IC14/1
  Gain10/1 -> IC15/1
  Gain11/1 -> IC16/1
  Gain12/1 -> IC17/1
  Gain13/1 -> IC19/1
  Gain14/1 -> IC18/1
  Gain15/1 -> IC24/1
  Gain16/1 -> IC25/1
  Gain17/1 -> IC20/1
  Gain18/1 -> IC21/1
  Gain19/1 -> IC22/1
  Gain20/1 -> IC23/1
  Demux/10 -> Gain10/1
  Demux/9 -> Gain9/1
  Demux/5 -> Gain1/1
  Demux/6 -> Gain6/1

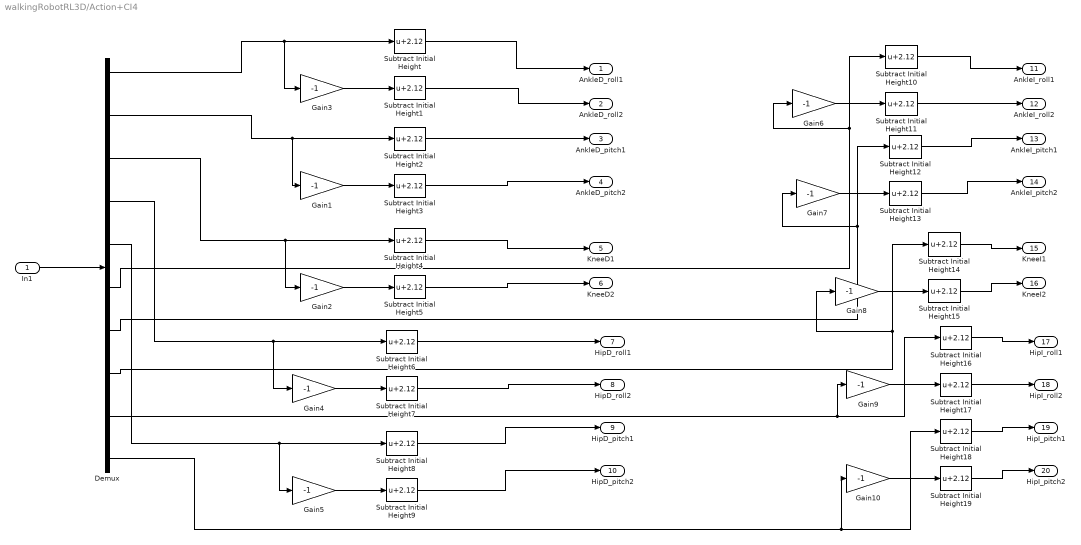
== system walkingRobotRL3D/Action+CI4 ==
  In1 : Inport
  Demux : Demux  Outputs=10
  Gain{1..10} (10 alike) : Gain  Gain=-1
  Subtract Initial Height{,1..19} (20 alike) : Bias  Bias=2.12
  AnkleD_roll1 : Outport
  AnkleD_roll2 : Outport  Port=2
  AnkleD_pitch1 : Outport  Port=3
  AnkleD_pitch2 : Outport  Port=4
  KneeD1 : Outport  Port=5
  KneeD2 : Outport  Port=6
  HipD_roll1 : Outport  Port=7
  HipD_roll2 : Outport  Port=8
  HipD_pitch1 : Outport  Port=9
  HipD_pitch2 : Outport  Port=10
  AnkleI_roll1 : Outport  Port=11
  AnkleI_roll2 : Outport  Port=12
  AnkleI_pitch1 : Outport  Port=13
  AnkleI_pitch2 : Outport  Port=14
  KneeI1 : Outport  Port=15
  KneeI2 : Outport  Port=16
  HipI_roll1 : Outport  Port=17
  HipI_roll2 : Outport  Port=18
  HipI_pitch1 : Outport  Port=19
  HipI_pitch2 : Outport  Port=20
  wires:
  In1/1 -> Demux/1
  Subtract Initial Height/1 -> AnkleD_roll1/1
  Demux/1 -> Gain3/1, Subtract Initial Height/1
  Subtract Initial Height1/1 -> AnkleD_roll2/1
  Gain3/1 -> Subtract Initial Height1/1
  Gain1/1 -> Subtract Initial Height3/1
  Demux/2 -> Gain1/1, Subtract Initial Height2/1
  Subtract Initial Height2/1 -> AnkleD_pitch1/1
  Subtract Initial Height3/1 -> AnkleD_pitch2/1
  Gain2/1 -> Subtract Initial Height5/1
  Demux/3 -> Gain2/1, Subtract Initial Height4/1
  Subtract Initial Height4/1 -> KneeD1/1
  Subtract Initial Height5/1 -> KneeD2/1
  Gain4/1 -> Subtract Initial Height7/1
  Demux/4 -> Subtract Initial Height6/1, Gain4/1
  Subtract Initial Height6/1 -> HipD_roll1/1
  Subtract Initial Height7/1 -> HipD_roll2/1
  Gain5/1 -> Subtract Initial Height9/1
  Demux/5 -> Gain5/1, Subtract Initial Height8/1
  Subtract Initial Height8/1 -> HipD_pitch1/1
  Subtract Initial Height9/1 -> HipD_pitch2/1
  Gain6/1 -> Subtract Initial Height11/1
  Subtract Initial Height10/1 -> AnkleI_roll1/1
  Subtract Initial Height11/1 -> AnkleI_roll2/1
  Demux/6 -> Gain6/1, Subtract Initial Height10/1
  Gain7/1 -> Subtract Initial Height13/1
  Subtract Initial Height12/1 -> AnkleI_pitch1/1
  Subtract Initial Height13/1 -> AnkleI_pitch2/1
  Demux/7 -> Gain7/1, Subtract Initial Height12/1
  Gain8/1 -> Subtract Initial Height15/1
  Subtract Initial Height14/1 -> KneeI1/1
  Subtract Initial Height15/1 -> KneeI2/1
  Demux/8 -> Gain8/1, Subtract Initial Height14/1
  Gain9/1 -> Subtract Initial Height17/1
  Subtract Initial Height16/1 -> HipI_roll1/1
  Subtract Initial Height17/1 -> HipI_roll2/1
  Demux/9 -> Gain9/1, Subtract Initial Height16/1
  Gain10/1 -> Subtract Initial Height19/1
  Subtract Initial Height18/1 -> HipI_pitch1/1
  Subtract Initial Height19/1 -> HipI_pitch2/1
  Demux/10 -> Gain10/1, Subtract Initial Height18/1

== system walkingRobotRL3D/Calculate Observation ==
  meas : Inport
  prevAct : Inport  Port=2
  Bus Selector : BusSelector  OutputSignals=Y,Z,VX,VY,VZ,yaw,pitch,roll,wx,wy,wz,measR.ankle_roll_angle,measR.ankle_roll_speed,measR.ankle_pitch_angle,measR.ankle_pitch_speed,measR.knee_angle,measR.knee_speed,measR.hip_roll_angle,measR.hip_roll_speed,measR.hip_pitch_angle,measR.hip_pitch_speed,measL.ankle_roll_angle,measL.ankle_roll_speed,measL.ankle_pitch_angle,measL.ankle_pitch_speed,measL.knee_angle,measL.knee_speed,measL.hip_roll_angle,measL.hip_roll_speed,measL.hip_pitch_angle,measL.hip_pitch_speed,measL.normal_force,measR.normal_force
  Compare To Zero : simulink/Logic and Bit Operations/Compare To Zero  relop=>  OutDataTypeStr=boolean
  Compare To Zero1 : simulink/Logic and Bit Operations/Compare To Zero  relop=>  OutDataTypeStr=boolean
  Data Type Conversion : DataTypeConversion
  Data Type Conversion1 : DataTypeConversion
  Mux : Mux  Inputs=34
  Rate Transition : RateTransition
  Scale Height : Gain  Gain=1/0.05
  Subtract Initial Height : Bias  Bias=-init_height/100
  observation : Outport  VectorParamsAs1DForOutWhenUnconnected=off
  wires:
  meas/1 -> Bus Selector/1
  Mux/1 -> Rate Transition/1
  Rate Transition/1 -> observation/1
  Bus Selector/2 -> Subtract Initial Height/1  "<Z>"
  Subtract Initial Height/1 -> Scale Height/1
  Scale Height/1 -> Mux/2  "Z_scaled"
  Bus Selector/1 -> Mux/1  "<Y>"
  Bus Selector/4 -> Mux/4  "<VY>"
  Bus Selector/3 -> Mux/3  "<VX>"
  Bus Selector/5 -> Mux/5  "<VZ>"
  Bus Selector/6 -> Mux/6  "<yaw>"
  Bus Selector/7 -> Mux/7  "<pitch>"
  Bus Selector/8 -> Mux/8  "<roll>"
  Bus Selector/9 -> Mux/9  "<wx>"
  Bus Selector/10 -> Mux/10  "<wy>"
  Bus Selector/11 -> Mux/11  "<wz>"
  Bus Selector/12 -> Mux/12  "<ankle_roll_angle>"
  Bus Selector/13 -> Mux/13  "<ankle_roll_speed>"
  Bus Selector/14 -> Mux/14  "<ankle_pitch_angle>"
  Bus Selector/15 -> Mux/15  "<ankle_pitch_speed>"
  Bus Selector/16 -> Mux/16  "<knee_angle>"
  Bus Selector/17 -> Mux/17  "<knee_speed>"
  Bus Selector/18 -> Mux/18  "<hip_roll_angle>"
  Bus Selector/19 -> Mux/19  "<hip_roll_speed>"
  Bus Selector/20 -> Mux/20  "<hip_pitch_angle>"
  Bus Selector/21 -> Mux/21  "<hip_pitch_speed>"
  Bus Selector/22 -> Mux/22  "<ankle_roll_angle>"
  Bus Selector/23 -> Mux/23  "<ankle_roll_speed>"
  Bus Selector/24 -> Mux/24  "<ankle_pitch_angle>"
  Bus Selector/25 -> Mux/25  "<ankle_pitch_speed>"
  Bus Selector/26 -> Mux/26  "<knee_angle>"
  Bus Selector/27 -> Mux/27  "<knee_speed>"
  Bus Selector/28 -> Mux/28  "<hip_roll_angle>"
  Bus Selector/29 -> Mux/29  "<hip_roll_speed>"
  Bus Selector/30 -> Mux/30  "<hip_pitch_angle>"
  Bus Selector/31 -> Mux/31  "<hip_pitch_speed>"
  prevAct/1 -> Mux/34
  Bus Selector/32 -> Compare To Zero/1  "<normal_force>"
  Bus Selector/33 -> Compare To Zero1/1  "<normal_force>"
  Compare To Zero/1 -> Data Type Conversion/1
  Compare To Zero1/1 -> Data Type Conversion1/1
  Data Type Conversion/1 -> Mux/32
  Data Type Conversion1/1 -> Mux/33

== system walkingRobotRL3D/Calculate Observation22 ==
  meas : Inport
  prevAct : Inport  Port=2
  Bus Selector : BusSelector  OutputSignals=Y,Z,VX,VY,VZ,yaw,pitch,roll,wx,wy,wz,measR.ankle_roll_angle,measR.ankle_roll_speed,measR.ankle_pitch_angle,measR.ankle_pitch_speed,measR.knee_angle,measR.knee_speed,measR.hip_roll_angle,measR.hip_roll_speed,measR.hip_pitch_angle,measR.hip_pitch_speed,measL.ankle_roll_angle,measL.ankle_roll_speed,measL.ankle_pitch_angle,measL.ankle_pitch_speed,measL.knee_angle,measL.knee_speed,measL.hip_roll_angle,measL.hip_roll_speed,measL.hip_pitch_angle,measL.hip_pitch_speed,measL.normal_force,measR.normal_force
  Compare To Zero : simulink/Logic and Bit Operations/Compare To Zero  relop=>  OutDataTypeStr=boolean
  Compare To Zero1 : simulink/Logic and Bit Operations/Compare To Zero  relop=>  OutDataTypeStr=boolean
  Data Type Conversion : DataTypeConversion
  Data Type Conversion1 : DataTypeConversion
  Mux : Mux  Inputs=34
  Rate Transition : RateTransition
  Scale Height : Gain  Gain=1/0.05
  Subtract Initial Height : Bias  Bias=-init_height/100
  observation : Outport  VectorParamsAs1DForOutWhenUnconnected=off
  wires:
  meas/1 -> Bus Selector/1
  Mux/1 -> Rate Transition/1
  Rate Transition/1 -> observation/1
  Bus Selector/2 -> Subtract Initial Height/1  "<Z>"
  Subtract Initial Height/1 -> Scale Height/1
  Scale Height/1 -> Mux/2  "Z_scaled"
  Bus Selector/1 -> Mux/1  "<Y>"
  Bus Selector/4 -> Mux/4  "<VY>"
  Bus Selector/3 -> Mux/3  "<VX>"
  Bus Selector/5 -> Mux/5  "<VZ>"
  Bus Selector/6 -> Mux/6  "<yaw>"
  Bus Selector/7 -> Mux/7  "<pitch>"
  Bus Selector/8 -> Mux/8  "<roll>"
  Bus Selector/9 -> Mux/9  "<wx>"
  Bus Selector/10 -> Mux/10  "<wy>"
  Bus Selector/11 -> Mux/11  "<wz>"
  Bus Selector/12 -> Mux/12  "<ankle_roll_angle>"
  Bus Selector/13 -> Mux/13  "<ankle_roll_speed>"
  Bus Selector/14 -> Mux/14  "<ankle_pitch_angle>"
  Bus Selector/15 -> Mux/15  "<ankle_pitch_speed>"
  Bus Selector/16 -> Mux/16  "<knee_angle>"
  Bus Selector/17 -> Mux/17  "<knee_speed>"
  Bus Selector/18 -> Mux/18  "<hip_roll_angle>"
  Bus Selector/19 -> Mux/19  "<hip_roll_speed>"
  Bus Selector/20 -> Mux/20  "<hip_pitch_angle>"
  Bus Selector/21 -> Mux/21  "<hip_pitch_speed>"
  Bus Selector/22 -> Mux/22  "<ankle_roll_angle>"
  Bus Selector/23 -> Mux/23  "<ankle_roll_speed>"
  Bus Selector/24 -> Mux/24  "<ankle_pitch_angle>"
  Bus Selector/25 -> Mux/25  "<ankle_pitch_speed>"
  Bus Selector/26 -> Mux/26  "<knee_angle>"
  Bus Selector/27 -> Mux/27  "<knee_speed>"
  Bus Selector/28 -> Mux/28  "<hip_roll_angle>"
  Bus Selector/29 -> Mux/29  "<hip_roll_speed>"
  Bus Selector/30 -> Mux/30  "<hip_pitch_angle>"
  Bus Selector/31 -> Mux/31  "<hip_pitch_speed>"
  prevAct/1 -> Mux/34
  Bus Selector/32 -> Compare To Zero/1  "<normal_force>"
  Bus Selector/33 -> Compare To Zero1/1  "<normal_force>"
  Compare To Zero/1 -> Data Type Conversion/1
  Compare To Zero1/1 -> Data Type Conversion1/1
  Data Type Conversion/1 -> Mux/32
  Data Type Conversion1/1 -> Mux/33

== system walkingRobotRL3D/Calculate Observation3 ==
  meas : Inport
  prevAct : Inport  Port=2
  Bus Selector : BusSelector  OutputSignals=Y,Z,VX,VY,VZ,yaw,pitch,roll,wx,wy,wz,measR.ankle_roll_angle,measR.ankle_roll_speed,measR.ankle_pitch_angle,measR.ankle_pitch_speed,measR.knee_angle,measR.knee_speed,measR.hip_roll_angle,measR.hip_roll_speed,measR.hip_pitch_angle,measR.hip_pitch_speed,measL.ankle_roll_angle,measL.ankle_roll_speed,measL.ankle_pitch_angle,measL.ankle_pitch_speed,measL.knee_angle,measL.knee_speed,measL.hip_roll_angle,measL.hip_roll_speed,measL.hip_pitch_angle,measL.hip_pitch_speed,measL.normal_force,measR.normal_force
  Compare To Zero : simulink/Logic and Bit Operations/Compare To Zero  relop=>  OutDataTypeStr=boolean
  Compare To Zero1 : simulink/Logic and Bit Operations/Compare To Zero  relop=>  OutDataTypeStr=boolean
  Data Type Conversion : DataTypeConversion
  Data Type Conversion1 : DataTypeConversion
  Mux : Mux  Inputs=34
  Rate Transition : RateTransition
  Scale Height : Gain  Gain=1/0.05
  Subtract Initial Height : Bias  Bias=-init_height/100
  observation : Outport  VectorParamsAs1DForOutWhenUnconnected=off
  wires:
  meas/1 -> Bus Selector/1
  Mux/1 -> Rate Transition/1
  Rate Transition/1 -> observation/1
  Bus Selector/2 -> Subtract Initial Height/1  "<Z>"
  Subtract Initial Height/1 -> Scale Height/1
  Scale Height/1 -> Mux/2  "Z_scaled"
  Bus Selector/1 -> Mux/1  "<Y>"
  Bus Selector/4 -> Mux/4  "<VY>"
  Bus Selector/3 -> Mux/3  "<VX>"
  Bus Selector/5 -> Mux/5  "<VZ>"
  Bus Selector/6 -> Mux/6  "<yaw>"
  Bus Selector/7 -> Mux/7  "<pitch>"
  Bus Selector/8 -> Mux/8  "<roll>"
  Bus Selector/9 -> Mux/9  "<wx>"
  Bus Selector/10 -> Mux/10  "<wy>"
  Bus Selector/11 -> Mux/11  "<wz>"
  Bus Selector/12 -> Mux/12  "<ankle_roll_angle>"
  Bus Selector/13 -> Mux/13  "<ankle_roll_speed>"
  Bus Selector/14 -> Mux/14  "<ankle_pitch_angle>"
  Bus Selector/15 -> Mux/15  "<ankle_pitch_speed>"
  Bus Selector/16 -> Mux/16  "<knee_angle>"
  Bus Selector/17 -> Mux/17  "<knee_speed>"
  Bus Selector/18 -> Mux/18  "<hip_roll_angle>"
  Bus Selector/19 -> Mux/19  "<hip_roll_speed>"
  Bus Selector/20 -> Mux/20  "<hip_pitch_angle>"
  Bus Selector/21 -> Mux/21  "<hip_pitch_speed>"
  Bus Selector/22 -> Mux/22  "<ankle_roll_angle>"
  Bus Selector/23 -> Mux/23  "<ankle_roll_speed>"
  Bus Selector/24 -> Mux/24  "<ankle_pitch_angle>"
  Bus Selector/25 -> Mux/25  "<ankle_pitch_speed>"
  Bus Selector/26 -> Mux/26  "<knee_angle>"
  Bus Selector/27 -> Mux/27  "<knee_speed>"
  Bus Selector/28 -> Mux/28  "<hip_roll_angle>"
  Bus Selector/29 -> Mux/29  "<hip_roll_speed>"
  Bus Selector/30 -> Mux/30  "<hip_pitch_angle>"
  Bus Selector/31 -> Mux/31  "<hip_pitch_speed>"
  prevAct/1 -> Mux/34
  Bus Selector/32 -> Compare To Zero/1  "<normal_force>"
  Bus Selector/33 -> Compare To Zero1/1  "<normal_force>"
  Compare To Zero/1 -> Data Type Conversion/1
  Compare To Zero1/1 -> Data Type Conversion1/1
  Data Type Conversion/1 -> Mux/32
  Data Type Conversion1/1 -> Mux/33

== system walkingRobotRL3D/Calculate Reward ==
  note: Ajustar el valor. 1 es muy grande, hace muy neg la funct reward...
  note: Each muscle which moves properly adds 1 and each one not moving properly subtracts one
  note: Reward function inspired by
      | "Emergence of Locomotion Behaviours in Rich Environments"
      | Google DeepMind, 2017
      | https://arxiv.org/pdf/1707.02286.pdf
  meas : Inport
  prevAct : Inport  Port=2
  Add1 : Sum
  Add2 : Sum  Inputs=+-+-
  Bus Selector : BusSelector  OutputSignals=VX,Y,Z
  Deviation Penalty Scaling Y : Gain  Gain=1.5
  Deviation Penalty Scaling Z : Gain  Gain=25
  Duration Reward : Constant  Value=25*Ts/Tf
  Forward Reward Scaling : Gain
  Individual Rewards : Scope  NumInputPorts=3
  Rate Transition : RateTransition  OutPortSampleTime=Ts
  Square1 : Math  Operator=square  SignedPower=on  SaturateOnIntegerOverflow=on
  Square3 : Math  Operator=square  SignedPower=on  SaturateOnIntegerOverflow=on
  Square4 : Math  Operator=square  SignedPower=on  SaturateOnIntegerOverflow=on
  Subtract Initial Height : Bias  Bias=-init_height/100
  Sum of Elements : Sum  Inputs=+
  Sum of Elements1 : Sum  Commented=on  Inputs=+
  Torque Penalty Scaling : Gain  Commented=on  Gain=0.01875
  Weight : Gain  Gain=0.02
  reward : Outport  VectorParamsAs1DForOutWhenUnconnected=off
  wires:
  Rate Transition/1 -> Bus Selector/1
  Add1/1 -> Add2/2, Individual Rewards/2  "deviation_penalty"
  Forward Reward Scaling/1 -> Add2/1, Individual Rewards/1  "forward_reward"
  Bus Selector/1 -> Forward Reward Scaling/1  "<VX>"
  Bus Selector/2 -> Square3/1  "<Y>"
  Square3/1 -> Deviation Penalty Scaling Y/1
  Square4/1 -> Deviation Penalty Scaling Z/1
  Bus Selector/3 -> Subtract Initial Height/1  "<Z>"
  Subtract Initial Height/1 -> Square4/1
  Deviation Penalty Scaling Y/1 -> Add1/1
  Duration Reward/1 -> Add2/3, Individual Rewards/3  "duration_reward"
  meas/1 -> Rate Transition/1
  Deviation Penalty Scaling Z/1 -> Add1/2
  Sum of Elements1/1 -> Torque Penalty Scaling/1
  Add2/1 -> reward/1
  Weight/1 -> Add2/4
  Sum of Elements/1 -> Weight/1
  Square1/1 -> Sum of Elements/1
  prevAct/1 -> Square1/1
